simulink model "motor_beam_model_sim"  (R2022b)
settings: Solver=VariableStepAuto  StartTime=0.0  StopTime=10.0  MaxStep=5.0E-5  RelTol=1e-3
values from neighbouring files (symbols this model uses):
  A = d_sys.A    [motor_beam_sim_main.m]
  Ac = [0, 1, 0, 0 ... (first row only)    [motor_beam_sim_main.m]
  B = d_sys.B    [motor_beam_sim_main.m]
  Bc = [0 0 0 k_v]'    [motor_beam_sim_main.m]
  C = d_sys.C    [motor_beam_sim_main.m]
  K = place(A,B,p_discrete)    [motor_beam_sim_main.m]
  L = place(A',C',po_discrete)'    [motor_beam_sim_main.m]
  OBS = 1    [motor_beam_sim_main.m]
  P_0 = 0*eye(4,4)    [motor_beam_sim_main.m]
  Q = 1e-10* eye(4)    [motor_beam_sim_main.m]
  R = diag([position_variance^2, angle_variance^2])    [motor_beam_sim_main.m]
  Ts = 1/fs    (= 0.01)    [motor_beam_sim_main.m]
undefined symbols (not defined in the file or in its folder): p_0, p_dot_0, p_dot_hat_0, p_hat_0, theta_0, theta_dot_0, theta_dot_hat_0, theta_hat_0
libraries: dspsrcs4 x3
settings Model: Creator=lucien  LastModifiedBy=lucien

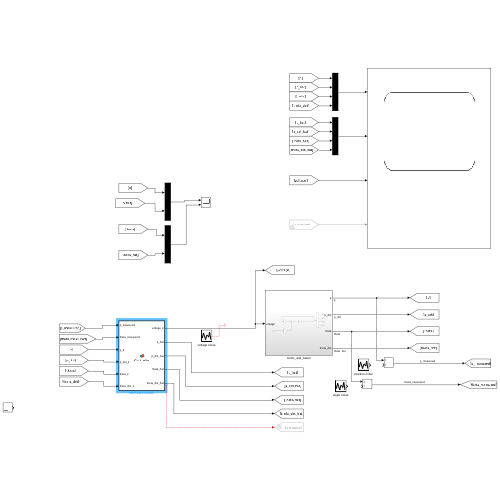
[thumbnail: Simulink's stored preview of the top-level diagram]
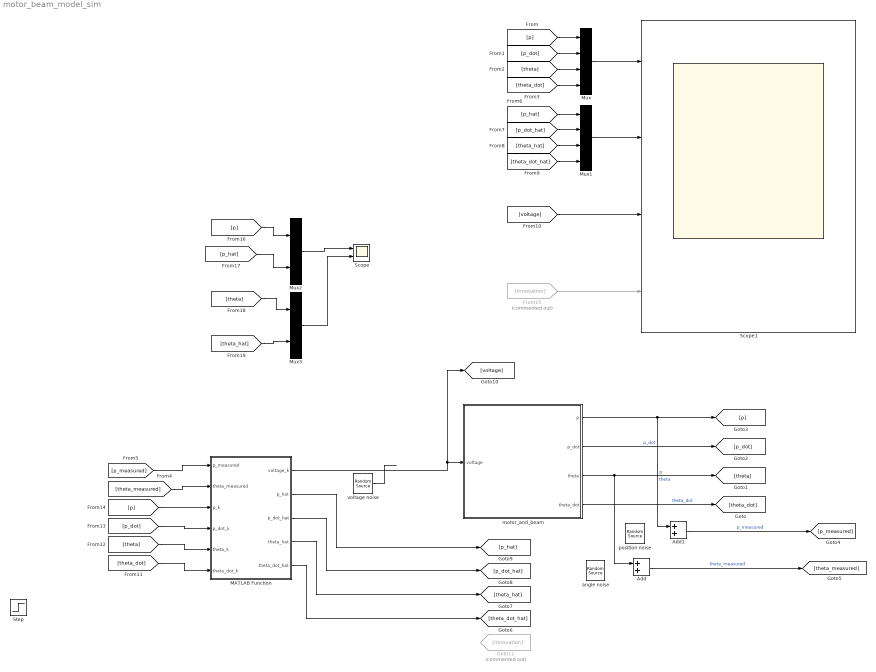
== system motor_beam_model_sim ==
  Add : Sum
  Add1 : Sum
  From15 : From  Commented=on  GotoTag=innovation
  Goto11 : Goto  Commented=on  GotoTag=innovation
  MATLAB Function : MATLAB Function  TreatAsAtomicUnit=on  SystemSampleTime=Ts
  Mux : Mux
  Mux1 : Mux
  Mux2 : Mux  Inputs=2
  Mux3 : Mux  Inputs=2
  Scope : Scope  NumInputPorts=2
  Scope1 : Scope  NumInputPorts=4
  Step : Step  SampleTime=0
  angle noise : dspsrcs4/Random Source  SrcType=Gaussian  NormMethod=Ziggurat  CltLength=12  MinVal=0  MaxVal=1  MeanVal=0  VarVal=angle_variance  RepMode=Not repeatable  rawSeed=1  IsInherit=off  SampMode=Discrete  SampTime=Ts  SampFrame=1  DataType=Double  OutComplex=Real  OutputFrames=off
  motor_and_beam : Subsystem
  position noise : dspsrcs4/Random Source  SrcType=Gaussian  NormMethod=Ziggurat  CltLength=12  MinVal=0  MaxVal=1  MeanVal=0  VarVal=position_variance  RepMode=Not repeatable  rawSeed=1  IsInherit=off  SampMode=Discrete  SampTime=Ts  SampFrame=1  DataType=Double  OutComplex=Real  OutputFrames=off
  voltage noise : dspsrcs4/Random Source  SrcType=Gaussian  NormMethod=Ziggurat  CltLength=12  MinVal=0  MaxVal=1  MeanVal=0  VarVal=voltage_noise  RepMode=Not repeatable  rawSeed=1  IsInherit=off  SampMode=Discrete  SampTime=Ts  SampFrame=1  DataType=Double  OutComplex=Real  OutputFrames=off
  wires:
  motor_and_beam/1(p) -> Add1/1, [p]  "p"
  motor_and_beam/3(theta) -> Add/1, [theta]  "theta"
  Add1/1 -> [p_measured]  "p_measured"
  Add/1 -> [theta_measured]  "theta_measured"
  [theta_measured] -> MATLAB Function/2(theta_measured)
  [p_measured] -> MATLAB Function/1(p_measured)
  MATLAB Function/2(p_hat) -> [p_hat]
  MATLAB Function/3(p_dot_hat) -> [p_dot_hat]
  MATLAB Function/4(theta_hat) -> [theta_hat]
  MATLAB Function/5(theta_dot_hat) -> [theta_dot_hat]
  motor_and_beam/2(p_dot) -> [p_dot]  "p_dot"
  motor_and_beam/4(theta_dot) -> [theta_dot]  "theta_dot"
  [p] -> Mux/1
  [p_dot] -> Mux/2
  [theta] -> Mux/3
  [theta_dot] -> Mux/4
  [p_hat] -> Mux1/1
  [p_dot_hat] -> Mux1/2
  [theta_hat] -> Mux1/3
  [theta_dot_hat] -> Mux1/4
  [voltage] -> Scope1/3
  Mux/1 -> Scope1/1
  Mux1/1 -> Scope1/2
  [p] -> MATLAB Function/3(p_k)
  [p_dot] -> MATLAB Function/4(p_dot_k)
  [theta] -> MATLAB Function/5(theta_k)
  [theta_dot] -> MATLAB Function/6(theta_dot_k)
  ? -> Goto11/1
  From15/1 -> Scope1/4
  voltage noise/1 -> ?
  MATLAB Function/1(voltage_k) -> [voltage], motor_and_beam/1(voltage)
  [p] -> Mux2/1
  [p_hat] -> Mux2/2
  Mux2/1 -> Scope/1
  [theta] -> Mux3/1
  [theta_hat] -> Mux3/2
  Mux3/1 -> Scope/2

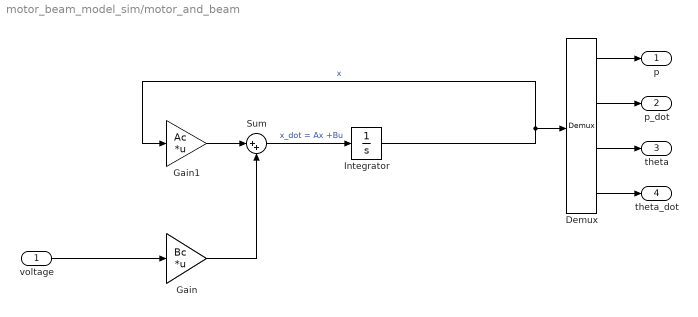
== system motor_beam_model_sim/motor_and_beam ==
  voltage : Inport
  Demux : Demux
  Gain : Gain  Gain=Bc  Multiplication=Matrix(K*u)
  Gain1 : Gain  Gain=Ac  Multiplication=Matrix(K*u)
  Integrator : Integrator  InitialCondition=[p_0,p_dot_0,theta_0,theta_dot_0]'
  Sum : Sum  Inputs=|++
  p : Outport
  p_dot : Outport  Port=2
  theta : Outport  Port=3
  theta_dot : Outport  Port=4
  wires:
  voltage/1 -> Gain/1
  Gain/1 -> Sum/2
  Sum/1 -> Integrator/1  "x_dot = Ax +Bu"
  Gain1/1 -> Sum/1
  Integrator/1 -> Demux/1, Gain1/1  "x"
  Demux/4 -> theta_dot/1
  Demux/3 -> theta/1
  Demux/2 -> p_dot/1
  Demux/1 -> p/1

== matlab function motor_beam_model_sim/MATLAB Function ==
  settings: updateMethod=DISCRETE  sampleTime=Ts
  data: p_measured input; theta_measured input; p_k input; p_dot_k input; theta_k input; theta_dot_k input; K parameter; voltage_k output; p_hat output; p_dot_hat output; theta_hat output; theta_dot_hat output; A parameter; B parameter; C parameter; Q parameter; R parameter; P_0 parameter; OBS parameter; p_hat_0 parameter; p_dot_hat_0 parameter; theta_hat_0 parameter; theta_dot_hat_0 parameter; L parameter
function [voltage_k, p_hat, p_dot_hat, theta_hat, theta_dot_hat] = Controller(p_measured,theta_measured, p_k, p_dot_k, theta_k, theta_dot_k, K, A, B, C, Q, R, P_0, OBS, p_hat_0, p_dot_hat_0, theta_hat_0, theta_dot_hat_0, L)
%% Initialise system and covaraince on first call
% persistent P_k 
% if isempty(P_k)
%     P_k = P_0;
% end

persistent x_hat_k 
if isempty(x_hat_k)
    x_hat_k = [p_hat_0, p_dot_hat_0, theta_hat_0, theta_dot_hat_0]'; %observer initialization x_hat(0) 
end

%% Control
% Desired setpoint
x_ref = [0, 0, 0, 0]';
% Desired reference to hold the setpoint
u_ref=0;
% calculate control action
if (OBS == 1)
    voltage_k=-K*(x_hat_k-x_ref)+u_ref;
else
    x_k = [p_k, p_dot_k, theta_k, theta_dot_k]';
    voltage_k=-K*(x_k-x_ref)+u_ref;
end
voltage_k = min(voltage_k, 12);
voltage_k = max(voltage_k, -12);

%% Observers
% construct the measurement vector
z_k = [p_measured, theta_measured]';

%% Kalman
% % predict
% % predict state forward
% x_hat_k_plus_1_priori = A * x_hat_k + B * voltage_k;
% % predict covaraince forward
% P_k_plus_1_priori = A * P_k * A' + Q;

% % update
% % compute kalman gain
% k_gain = P_k_plus_1_priori * C' / (C*P_k_plus_1_priori*C'+R);
% % predict measurement for predicted state
% measurement_predict = C * x_hat_k_plus_1_priori;
% % update and correct estimate for x_hat
% innovation = z_k - measurement_predict;
% x_hat_k_plus_1 = x_hat_k_plus_1_priori + k_gain*(innovation);
% % update and correct estimate for covariance
% P_k = (eye(4,4) - k_gain * C) * P_k_plus_1_priori;
% x_hat_k = A * x_hat_k + B * voltage_k + k_gain * innovation;

%% Luenberger
x_hat_k = A * x_hat_k + B * voltage_k +L * (z_k - C*x_hat_k);

%% Output current estimates
p_hat = x_hat_k(1);
p_dot_hat = x_hat_k(2);
theta_hat = x_hat_k(3);
theta_dot_hat = x_hat_k(4);

end
